simulink model "MBD2_problem4"  (R2020b)
settings: Solver=VariableStepAuto  StartTime=0.0  StopTime=0.2  RelTol=1e-3
InitFcn:
  | J=3.2284e-6;
  | b=3.5077e-6;
  | Ke= 0.0274;
  | Kt=   0.0274;
  | R=4;
  | L=2.75e-6;
settings Model: Creator=Lenovo  LastModifiedBy=Lenovo

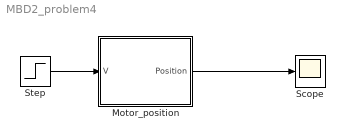
== system MBD2_problem4 ==
  Motor_position : Subsystem
  Scope : Scope
  Step : Step  Time=0  After=5  SampleTime=0
  wires:
  Step/1 -> Motor_position/1(V)
  Motor_position/1(Position) -> Scope/1

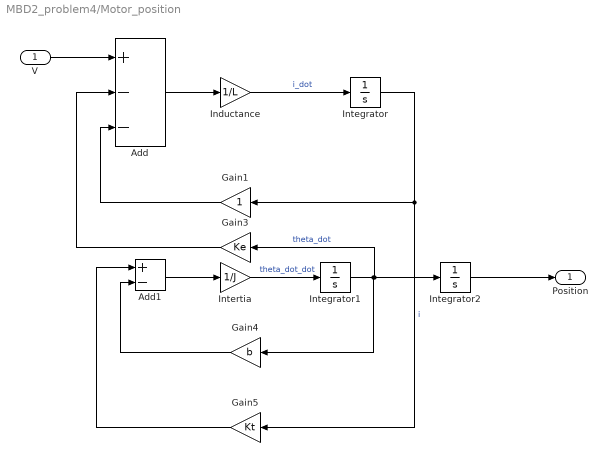
== system MBD2_problem4/Motor_position ==
  V : Inport
  Add : Sum  Inputs=+--
  Add1 : Sum  Inputs=+-
  Gain1 : Gain
  Gain3 : Gain  Gain=Ke
  Gain4 : Gain  Gain=b
  Gain5 : Gain  Gain=Kt
  Inductance : Gain  Gain=1/L
  Integrator : Integrator
  Integrator1 : Integrator
  Integrator2 : Integrator
  Intertia : Gain  Gain=1/J
  Position : Outport
  wires:
  Integrator1/1 -> Integrator2/1, Gain3/1, Gain4/1  "theta_dot"
  Gain1/1 -> Add/3
  Intertia/1 -> Integrator1/1  "theta_dot_dot"
  Gain3/1 -> Add/2
  Integrator2/1 -> Position/1
  Add/1 -> Inductance/1
  Gain4/1 -> Add1/2
  Add1/1 -> Intertia/1
  Integrator/1 -> Gain1/1, Gain5/1  "i"
  Gain5/1 -> Add1/1
  Inductance/1 -> Integrator/1  "i_dot"
  V/1 -> Add/1
